simulink model "chris_3R_setpoint"  (R2024b)
settings: Solver=FixedStepDiscrete  StartTime=0.0  StopTime=3  FixedStep=0.1  MaxStep=0.1  RelTol=1e-3
libraries: simulink x1, realtime_pacer_lib x1
settings Model: Creator=RSL  LastModifiedBy=cwaight
settings SolverCC: AlgebraicLoopSolver=TrustRegion
settings DataIOCC: ReturnWorkspaceOutputs=off
settings DebuggingCC: UnconnectedInputMsg=warning  UnconnectedOutputMsg=warning  UnconnectedLineMsg=warning  ArithmeticOperatorsInVariantConditions=warning
settings ModelReferenceCC: EnableRefExpFcnMdlSchedulingChecks=on
settings SFSimCC: SimUseLocalCustomCode=off  CustomCodeUndefinedFunction=UseInterfaceOnly
settings RTWCC: RTWUseLocalCustomCode=off  GPUComputeCapability=3.5
settings CodeAppCC: StateflowObjectComments=on

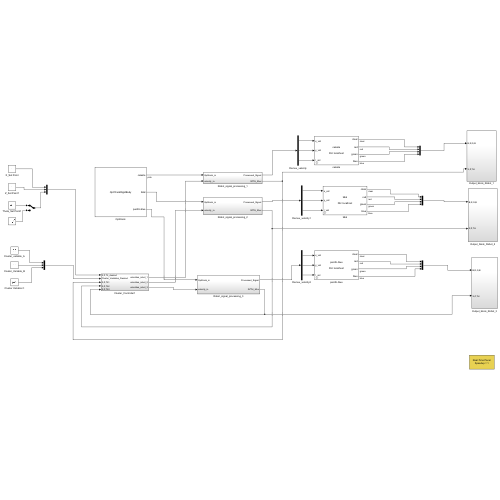
[thumbnail: Simulink's stored preview of the top-level diagram]
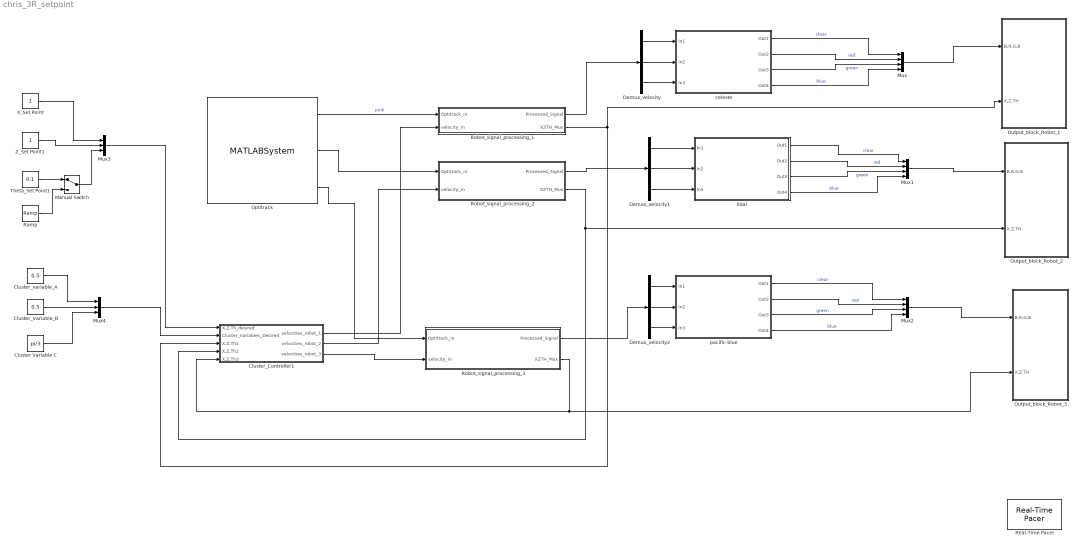
== system chris_3R_setpoint ==
  Cluster Variable C : Constant  Value=pi/3
  Cluster_Controller1 : Subsystem
  Cluster_Variable_B : Constant  Value=0.5
  Cluster_variable_A : Constant  Value=0.5
  Demux_velocity : Demux  Outputs=3
  Demux_velocity1 : Demux  Outputs=3
  Demux_velocity2 : Demux  Outputs=3
  Manual Switch : ManualSwitch
  Mux : Mux
  Mux1 : Mux
  Mux2 : Mux
  Mux3 : Mux  Inputs=3
  Mux4 : Mux  Inputs=3
  Optitrack : MATLABSystem  System=OptiTrackRigidBody  coordinateTransformationMatrix=[ 1, 0, 0; 0, 0, 1; 0, -1, 0 ]  rigidBodyNames={ 'celeste','tidal','pacific-blue'}  orientationFormat=Euler angles  debug=on  natNetHostAddress=127.0.0.1  natNetClientAddress=127.0.0.1  dllPath=C:\DecaMATLAB\NatNetSDK\lib\x64\NatNetML.dll  unicast=off
      mask Type: OptiTrackRigidBody
      mask Display:
      | disp('OptiTrackRigidBody');
      | port_label('output',1,'celeste');
      | port_label('output',2,'tidal');
      | port_label('output',3,'pacific-blue');
  Output_block_Robot_1 : Subsystem
  Output_block_Robot_2 : Subsystem
  Output_block_Robot_3 : Subsystem
  Ramp : simulink/Sources/Ramp  slope=1  start=0  InitialOutput=0.1
  Real-Time Pacer : realtime_pacer_lib/Real-Time Pacer  simTimePerRealTime=1
  Robot_signal_processing_1 : Subsystem
  Robot_signal_processing_2 : Subsystem
  Robot_signal_processing_3 : Subsystem
  "Theta_Set Point1 " : Constant  Value=0.1
  X_Set Point : Constant
  Z_Set Point1 : Constant
  celeste : Subsystem  mask(DecabotMask){robotName=celeste, decabotHelper=localhost, robotAddress=, useDataTurbine=off, useDirectSocket=on, debug=off}
      mask prompts: robotName "Robot name:"; decabotHelper "DecabotHelper/DataTurbine server:"; robotAddress "Robot network address (optional):"; useDataTurbine "Use DataTurbine"; useDirectSocket "Use direct robot TCP connection"; debug "Log debug messages"
      mask help: This is a masked subsystem that contains a Decabot block for bidirectional communication with a decabot over a direct TCP socket connection.
      mask init:
      | robotName = 'Nobody';
      | decabotHelper = 'localhost';
      | robotAddress = '';
      | useDataTurbine = true;
      | debug = true;
      mask TypeOptions robotName: decabot/robotName
      mask Callback robotName:
      | try
      |     set_param( gcb( ), 'Name', get_param( gcb( ), 'robotName' ) );
      | end
      mask TypeOptions decabotHelper: decabot/decabotHelper
      mask TypeOptions robotAddress: decabot/robotAddress
      mask TypeOptions useDataTurbine: decabot/useDataTurbine
      mask TypeOptions useDirectSocket: decabot/useDirectSocket
      mask TypeOptions debug: decabot/debug
      mask Display:
      | disp( [get_param( gcb( ), 'robotName' ) '\n\nDH: ' get_param( gcb( ), 'decabotHelper' ) ] );
      | 
      | port_label('input',1,'x_vel');
      | port_label('input',2,'y_vel');
      | port_label('input',3,'t_vel');
      | 
      | port_label('output',1,'clear');
      | port_label('output',2,'red');
      | port_label('output',3,'green');
      | port_label('output',4,'blue');
  pacific-blue : Subsystem  mask(DecabotMask){robotName=pacific-blue, decabotHelper=localhost, robotAddress=, useDataTurbine=off, useDirectSocket=on, debug=off}
      mask prompts: robotName "Robot name:"; decabotHelper "DecabotHelper/DataTurbine server:"; robotAddress "Robot network address (optional):"; useDataTurbine "Use DataTurbine"; useDirectSocket "Use direct robot TCP connection"; debug "Log debug messages"
      mask help: This is a masked subsystem that contains a Decabot block for bidirectional communication with a decabot over a direct TCP socket connection.
      mask init:
      | robotName = 'Nobody';
      | decabotHelper = 'localhost';
      | robotAddress = '';
      | useDataTurbine = true;
      | debug = true;
      mask TypeOptions robotName: decabot/robotName
      mask Callback robotName:
      | try
      |     set_param( gcb( ), 'Name', get_param( gcb( ), 'robotName' ) );
      | end
      mask TypeOptions decabotHelper: decabot/decabotHelper
      mask TypeOptions robotAddress: decabot/robotAddress
      mask TypeOptions useDataTurbine: decabot/useDataTurbine
      mask TypeOptions useDirectSocket: decabot/useDirectSocket
      mask TypeOptions debug: decabot/debug
      mask Display:
      | disp( [get_param( gcb( ), 'robotName' ) '\n\nDH: ' get_param( gcb( ), 'decabotHelper' ) ] );
      | 
      | port_label('input',1,'x_vel');
      | port_label('input',2,'y_vel');
      | port_label('input',3,'t_vel');
      | 
      | port_label('output',1,'clear');
      | port_label('output',2,'red');
      | port_label('output',3,'green');
      | port_label('output',4,'blue');
  tidal : Subsystem  mask(DecabotMask){robotName=tidal, decabotHelper=localhost, robotAddress=, useDataTurbine=off, useDirectSocket=on, debug=off}
      mask prompts: robotName "Robot name:"; decabotHelper "DecabotHelper/DataTurbine server:"; robotAddress "Robot network address (optional):"; useDataTurbine "Use DataTurbine"; useDirectSocket "Use direct robot TCP connection"; debug "Log debug messages"
      mask help: This is a masked subsystem that contains a Decabot block for bidirectional communication with a decabot over a direct TCP socket connection.
      mask init:
      | robotName = 'Nobody';
      | decabotHelper = 'localhost';
      | robotAddress = '';
      | useDataTurbine = true;
      | debug = true;
      mask TypeOptions robotName: decabot/robotName
      mask Callback robotName:
      | try
      |     set_param( gcb( ), 'Name', get_param( gcb( ), 'robotName' ) );
      | end
      mask TypeOptions decabotHelper: decabot/decabotHelper
      mask TypeOptions robotAddress: decabot/robotAddress
      mask TypeOptions useDataTurbine: decabot/useDataTurbine
      mask TypeOptions useDirectSocket: decabot/useDirectSocket
      mask TypeOptions debug: decabot/debug
      mask Display:
      | disp( [get_param( gcb( ), 'robotName' ) '\n\nDH: ' get_param( gcb( ), 'decabotHelper' ) ] );
      | 
      | port_label('input',1,'x_vel');
      | port_label('input',2,'y_vel');
      | port_label('input',3,'t_vel');
      | 
      | port_label('output',1,'clear');
      | port_label('output',2,'red');
      | port_label('output',3,'green');
      | port_label('output',4,'blue');
  wires:
  Demux_velocity/3 -> celeste/3(In3)
  Demux_velocity/1 -> celeste/1(In1)
  Demux_velocity/2 -> celeste/2(In2)
  X_Set Point/1 -> Mux3/1
  Optitrack/1 -> Robot_signal_processing_1/1(Optitrack_in)  "pink"
  Robot_signal_processing_1/1(Processed_Signal) -> Demux_velocity/1
  celeste/1(Out1) -> Mux/1  "clear"
  celeste/2(Out2) -> Mux/2  "red"
  celeste/3(Out3) -> Mux/3  "green"
  celeste/4(Out4) -> Mux/4  "blue"
  Robot_signal_processing_1/2(XZTH_Mux) -> Output_block_Robot_1/2(X,Z,TH), Cluster_Controller1/3(X,Z,Th1)
  Mux/1 -> Output_block_Robot_1/1(B,R,G,B)
  Demux_velocity1/3 -> tidal/3(In3)
  Demux_velocity1/1 -> tidal/1(In1)
  Demux_velocity1/2 -> tidal/2(In2)
  Robot_signal_processing_2/1(Processed_Signal) -> Demux_velocity1/1
  tidal/1(Out1) -> Mux1/1  "clear"
  tidal/2(Out2) -> Mux1/2  "red"
  tidal/3(Out3) -> Mux1/3  "green"
  tidal/4(Out4) -> Mux1/4  "blue"
  Mux1/1 -> Output_block_Robot_2/1(B,R,G,B)
  Demux_velocity2/3 -> pacific-blue/3(In3)
  Demux_velocity2/1 -> pacific-blue/1(In1)
  Demux_velocity2/2 -> pacific-blue/2(In2)
  Robot_signal_processing_3/1(Processed_Signal) -> Demux_velocity2/1
  pacific-blue/1(Out1) -> Mux2/1  "clear"
  pacific-blue/2(Out2) -> Mux2/2  "red"
  pacific-blue/3(Out3) -> Mux2/3  "green"
  pacific-blue/4(Out4) -> Mux2/4  "blue"
  Mux2/1 -> Output_block_Robot_3/1(B,R,G,B)
  Robot_signal_processing_3/2(XZTH_Mux) -> Output_block_Robot_3/2(X,Z,TH), Cluster_Controller1/5(X,Z,Th3)
  Optitrack/2 -> Robot_signal_processing_2/1(Optitrack_in)
  Optitrack/3 -> Robot_signal_processing_3/1(Optitrack_in)
  Cluster_Controller1/1(velocities_robot_1) -> Robot_signal_processing_1/2(velocity_in)
  Z_Set Point1/1 -> Mux3/2
  Cluster_Controller1/3(velocities_robot_3) -> Robot_signal_processing_3/2(velocity_in)
  Mux3/1 -> Cluster_Controller1/1(X,Z,Th_desired)
  Cluster_Controller1/2(velocities_robot_2) -> Robot_signal_processing_2/2(velocity_in)
  Cluster_variable_A/1 -> Mux4/1
  Cluster_Variable_B/1 -> Mux4/2
  Cluster Variable C/1 -> Mux4/3
  Mux4/1 -> Cluster_Controller1/2(Cluster_Variables_Desired)
  Robot_signal_processing_2/2(XZTH_Mux) -> Cluster_Controller1/4(X,Z,Th2), Output_block_Robot_2/2(X,Z,TH)
  Ramp/1 -> Manual Switch/2
  "Theta_Set Point1 "/1 -> Manual Switch/1
  Manual Switch/1 -> Mux3/3

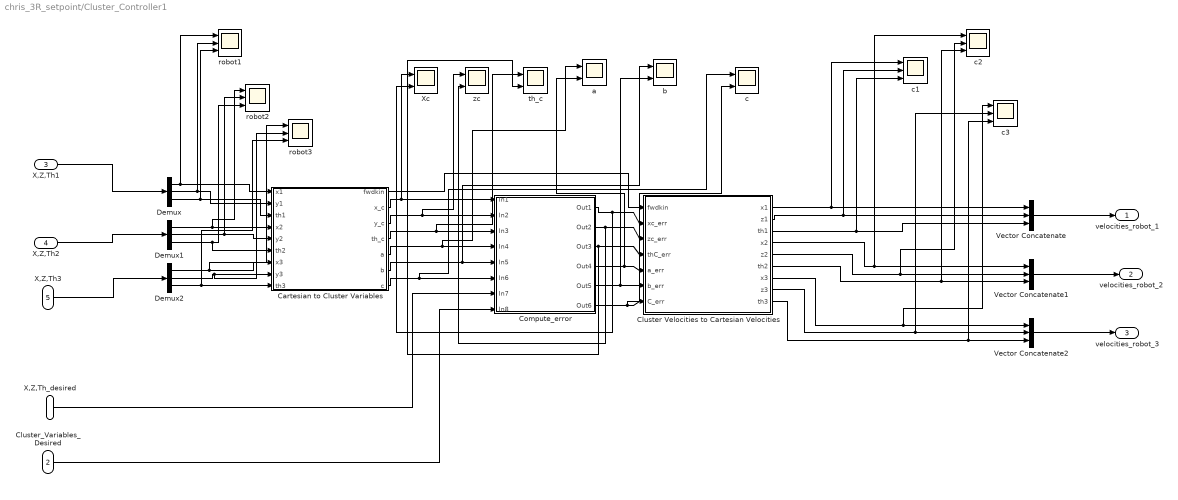
== system chris_3R_setpoint/Cluster_Controller1 ==
  X,Z,Th_desired : Inport
  Cluster_Variables_Desired : Inport  Port=2
  X,Z,Th1 : Inport  Port=3
  X,Z,Th2 : Inport  Port=4
  X,Z,Th3 : Inport  Port=5
  Cartesian to Cluster Variables : MATLAB Function  TreatAsAtomicUnit=on
  Cluster Velocities to Cartesian Velocities : MATLAB Function  TreatAsAtomicUnit=on
  Compute_error : Subsystem
  Demux : Demux  Outputs=3
  Demux1 : Demux  Outputs=3
  Demux2 : Demux  Outputs=3
  Vector Concatenate : Concatenate  NumInputs=3
  Vector Concatenate1 : Concatenate  NumInputs=3
  Vector Concatenate2 : Concatenate  NumInputs=3
  Xc : Scope  NumInputPorts=2
  a : Scope  NumInputPorts=2
  b : Scope  NumInputPorts=2
  c : Scope  NumInputPorts=2
  c1 : Scope  NumInputPorts=3
  c2 : Scope  NumInputPorts=3
  c3 : Scope  NumInputPorts=3
  robot1 : Scope  NumInputPorts=3
  robot2 : Scope  NumInputPorts=3
  robot3 : Scope  NumInputPorts=3
  th_c : Scope  NumInputPorts=2
  zc : Scope  NumInputPorts=2
  velocities_robot_1 : Outport
  velocities_robot_2 : Outport  Port=2
  velocities_robot_3 : Outport  Port=3
  wires:
  X,Z,Th1/1 -> Demux/1
  X,Z,Th2/1 -> Demux1/1
  X,Z,Th3/1 -> Demux2/1
  Vector Concatenate/1 -> velocities_robot_1/1
  Cluster Velocities to Cartesian Velocities/2(z1) -> c1/2, Vector Concatenate/2
  Cluster Velocities to Cartesian Velocities/1(x1) -> c1/1, Vector Concatenate/1
  Vector Concatenate1/1 -> velocities_robot_2/1
  Cluster Velocities to Cartesian Velocities/5(z2) -> c2/2, Vector Concatenate1/2
  Cluster Velocities to Cartesian Velocities/4(x2) -> c2/1, Vector Concatenate1/1
  Vector Concatenate2/1 -> velocities_robot_3/1
  Cluster Velocities to Cartesian Velocities/8(z3) -> c3/2, Vector Concatenate2/2
  Cluster Velocities to Cartesian Velocities/7(x3) -> c3/1, Vector Concatenate2/1
  Demux/1 -> robot1/1, Cartesian to Cluster Variables/1(x1)
  Demux/2 -> robot1/2, Cartesian to Cluster Variables/2(y1)
  Demux/3 -> robot1/3, Cartesian to Cluster Variables/3(th1)
  Demux1/1 -> robot2/1, Cartesian to Cluster Variables/4(x2)
  Demux1/2 -> robot2/2, Cartesian to Cluster Variables/5(y2)
  Demux1/3 -> robot2/3, Cartesian to Cluster Variables/6(th2)
  Demux2/1 -> robot3/1, Cartesian to Cluster Variables/7(x3)
  Demux2/2 -> robot3/2, Cartesian to Cluster Variables/8(y3)
  Demux2/3 -> robot3/3, Cartesian to Cluster Variables/9(th3)
  Cartesian to Cluster Variables/2(x_c) -> Xc/1, Compute_error/1(In1)
  Cartesian to Cluster Variables/3(y_c) -> zc/1, Compute_error/2(In2)
  Cartesian to Cluster Variables/4(th_c) -> th_c/1, Compute_error/3(In3)
  Cartesian to Cluster Variables/5(a) -> a/1, Compute_error/4(In4)
  Cartesian to Cluster Variables/6(b) -> b/1, Compute_error/5(In5)
  Cartesian to Cluster Variables/7(c) -> c/1, Compute_error/6(In6)
  X,Z,Th_desired/1 -> Compute_error/7(In7)
  Cluster_Variables_Desired/1 -> Compute_error/8(In8)
  Compute_error/1(Out1) -> Xc/2, Cluster Velocities to Cartesian Velocities/2(xc_err)
  Compute_error/2(Out2) -> zc/2, Cluster Velocities to Cartesian Velocities/3(zc_err)
  Compute_error/3(Out3) -> th_c/2, Cluster Velocities to Cartesian Velocities/4(thC_err)
  Compute_error/4(Out4) -> a/2, Cluster Velocities to Cartesian Velocities/5(a_err)
  Compute_error/5(Out5) -> b/2, Cluster Velocities to Cartesian Velocities/6(b_err)
  Compute_error/6(Out6) -> c/2, Cluster Velocities to Cartesian Velocities/7(C_err)
  Cartesian to Cluster Variables/1(fwdkin) -> Cluster Velocities to Cartesian Velocities/1(fwdkin)
  Cluster Velocities to Cartesian Velocities/3(th1) -> c1/3, Vector Concatenate/3
  Cluster Velocities to Cartesian Velocities/6(th2) -> c2/3, Vector Concatenate1/3
  Cluster Velocities to Cartesian Velocities/9(th3) -> c3/3, Vector Concatenate2/3

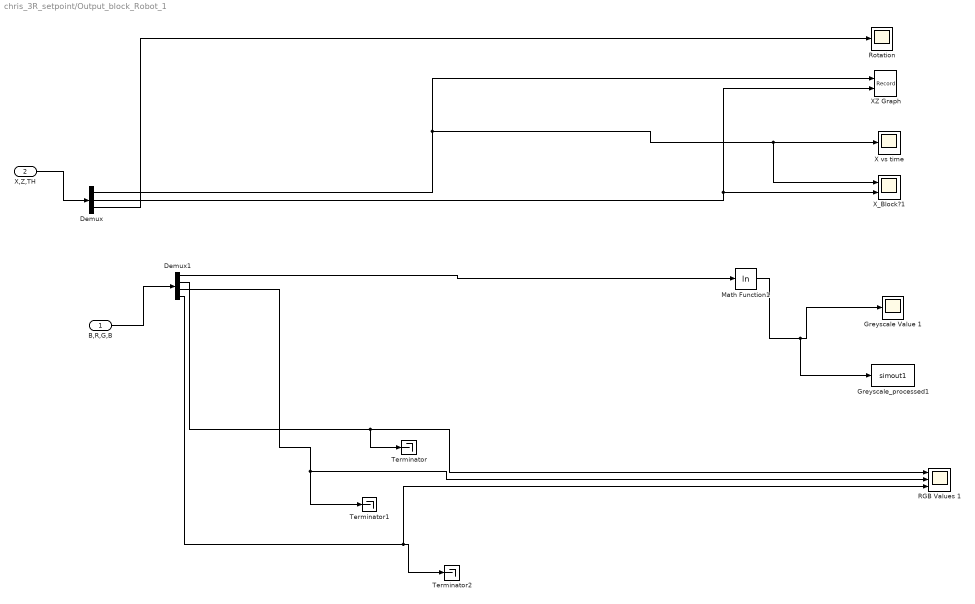
== system chris_3R_setpoint/Output_block_Robot_1 ==
  B,R,G,B : Inport
  X,Z,TH : Inport  Port=2
  " Greyscale_processed1" : ToWorkspace  VariableName=simout1  SaveFormat=Timeseries  SampleTime=-1
  Demux : Demux  Outputs=3
  Demux1 : Demux
  Greyscale Value 1 : Scope
  Math Function1 : Math  Operator=log  SignedPower=on
  "RGB Values 1 " : Scope  NumInputPorts=3
  Rotation : Scope
  Terminator : Terminator
  Terminator1 : Terminator
  Terminator2 : Terminator
  X vs time : Scope
  XZ Graph : Record  FileSettingsInternal="{\"entries\":[{\"content\":{\"excelSettings\":{\"content\":{},\"type\":\"Streamout.ExcelSettings\"}},\"type\":\"Streamout.FileSettingStorage\",\"uuid\":\"\"}],\"packageUris\":[\"http:\\/\\/schema.mathworks.com\\/mf0\\/streamout_blocks\\/R2020a\"],\"version\":\"1.0\"}"  Layout=[1 1]  SignalsInternal="{\"entries\":[{\"content\":{\"signals\":[{\"content\":{\"blockPath\":[],\"dimensions\":[1],\"domain\":\"\",\"lineColor\":\"#a2142f\",\"plots\":[ 1 ],\"port\":1,\"sid\":[\"\"],\"signalID\":1,\"signalName\":\"Demux:1\"},\"type\":\"RecordBlkView.Signal\",\"uuid\":\"\"},{\"content\":{\"blockPath\":[],\"dimensions\":[1],\"domain\":\"\",\"lineColor\":\"#139fff\",\"plots\":[ 1 ],\"port\":2,\"sid\":[\"\"],\"signalID\":2,\"signalName\":\"Demux:2\"},\"type\":\"RecordBlkView.Signal\",\"uuid\":\"\"}]},\"type\":\"RecordBlkView.InputSignals\",\"uuid\":\"\"}],\"packageUris\":[\"http:\\/\\/schema.mathworks.com\\/mf0\\/streamout_blocks\\/R2020a\"],\"version\":\"1.0\"}"  VisualizationBindings="{\"xyplotplugin\":{\"info\":[{\"series\":[{\"bindingParametersList\":[{\"parameter\":\"X-Axis\",\"signalID\":1,\"signalName\":\"Demux:1\"},{\"parameter\":\"Y-Axis\",\"signalID\":2,\"signalName\":\"Demux:2\"}],\"seriesID\":0}],\"subplotID\":1}]}}"  CompatibilityTag=XY  st=-1
  X_Block?1 : Scope  NumInputPorts=2
  wires:
  Demux/3 -> Rotation/1
  Demux/2 -> XZ Graph/2, X_Block?1/2
  Demux1/2 -> "RGB Values 1 "/1, Terminator/1
  Demux1/4 -> "RGB Values 1 "/3, Terminator2/1
  Math Function1/1 -> " Greyscale_processed1"/1, Greyscale Value 1/1
  Demux1/3 -> Terminator1/1, "RGB Values 1 "/2
  X,Z,TH/1 -> Demux/1
  Demux/1 -> X_Block?1/1, X vs time/1, XZ Graph/1
  Demux1/1 -> Math Function1/1
  B,R,G,B/1 -> Demux1/1

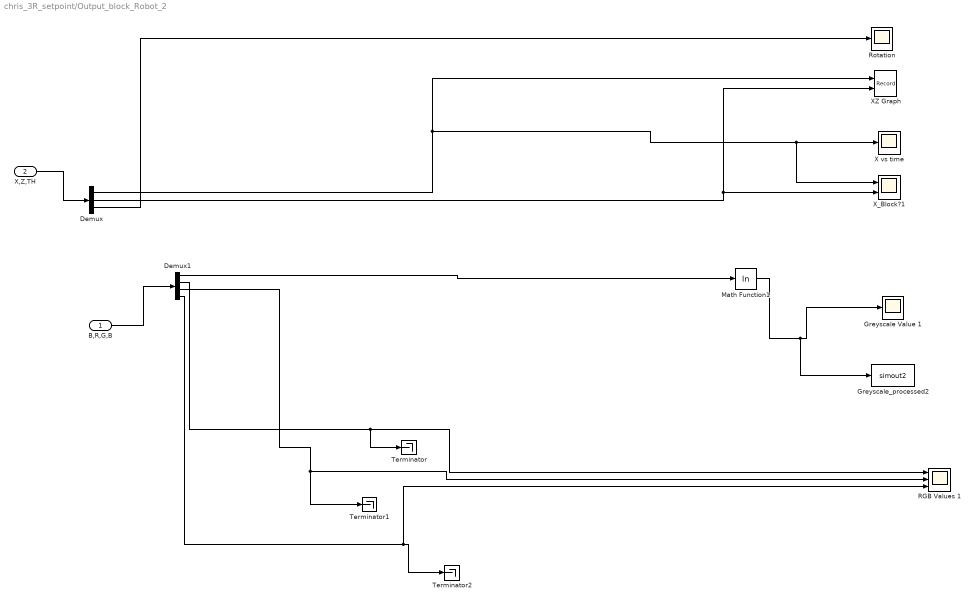
== system chris_3R_setpoint/Output_block_Robot_2 ==
  B,R,G,B : Inport
  X,Z,TH : Inport  Port=2
  " Greyscale_processed2" : ToWorkspace  VariableName=simout2  SaveFormat=Timeseries  SampleTime=-1
  Demux : Demux  Outputs=3
  Demux1 : Demux
  Greyscale Value 1 : Scope
  Math Function1 : Math  Operator=log  SignedPower=on
  "RGB Values 1 " : Scope  NumInputPorts=3
  Rotation : Scope
  Terminator : Terminator
  Terminator1 : Terminator
  Terminator2 : Terminator
  X vs time : Scope
  XZ Graph : Record  FileSettingsInternal="{\"entries\":[{\"content\":{\"excelSettings\":{\"content\":{},\"type\":\"Streamout.ExcelSettings\"}},\"type\":\"Streamout.FileSettingStorage\",\"uuid\":\"\"}],\"packageUris\":[\"http:\\/\\/schema.mathworks.com\\/mf0\\/streamout_blocks\\/R2020a\"],\"version\":\"1.0\"}"  Layout=[1 1]  SignalsInternal="{\"entries\":[{\"content\":{\"signals\":[{\"content\":{\"blockPath\":[],\"dimensions\":[1],\"domain\":\"\",\"lineColor\":\"#a2142f\",\"plots\":[ 1 ],\"port\":1,\"sid\":[\"\"],\"signalID\":1,\"signalName\":\"Demux:1\"},\"type\":\"RecordBlkView.Signal\",\"uuid\":\"\"},{\"content\":{\"blockPath\":[],\"dimensions\":[1],\"domain\":\"\",\"lineColor\":\"#139fff\",\"plots\":[ 1 ],\"port\":2,\"sid\":[\"\"],\"signalID\":2,\"signalName\":\"Demux:2\"},\"type\":\"RecordBlkView.Signal\",\"uuid\":\"\"}]},\"type\":\"RecordBlkView.InputSignals\",\"uuid\":\"\"}],\"packageUris\":[\"http:\\/\\/schema.mathworks.com\\/mf0\\/streamout_blocks\\/R2020a\"],\"version\":\"1.0\"}"  VisualizationBindings="{\"xyplotplugin\":{\"info\":[{\"series\":[{\"bindingParametersList\":[{\"parameter\":\"X-Axis\",\"signalID\":1,\"signalName\":\"Demux:1\"},{\"parameter\":\"Y-Axis\",\"signalID\":2,\"signalName\":\"Demux:2\"}],\"seriesID\":0}],\"subplotID\":1}]}}"  CompatibilityTag=XY  st=-1
  X_Block?1 : Scope  NumInputPorts=2
  wires:
  Demux/3 -> Rotation/1
  Demux/2 -> XZ Graph/2, X_Block?1/2
  Demux1/2 -> "RGB Values 1 "/1, Terminator/1
  Demux1/4 -> "RGB Values 1 "/3, Terminator2/1
  Math Function1/1 -> " Greyscale_processed2"/1, Greyscale Value 1/1
  Demux1/3 -> Terminator1/1, "RGB Values 1 "/2
  X,Z,TH/1 -> Demux/1
  Demux/1 -> X_Block?1/1, X vs time/1, XZ Graph/1
  Demux1/1 -> Math Function1/1
  B,R,G,B/1 -> Demux1/1

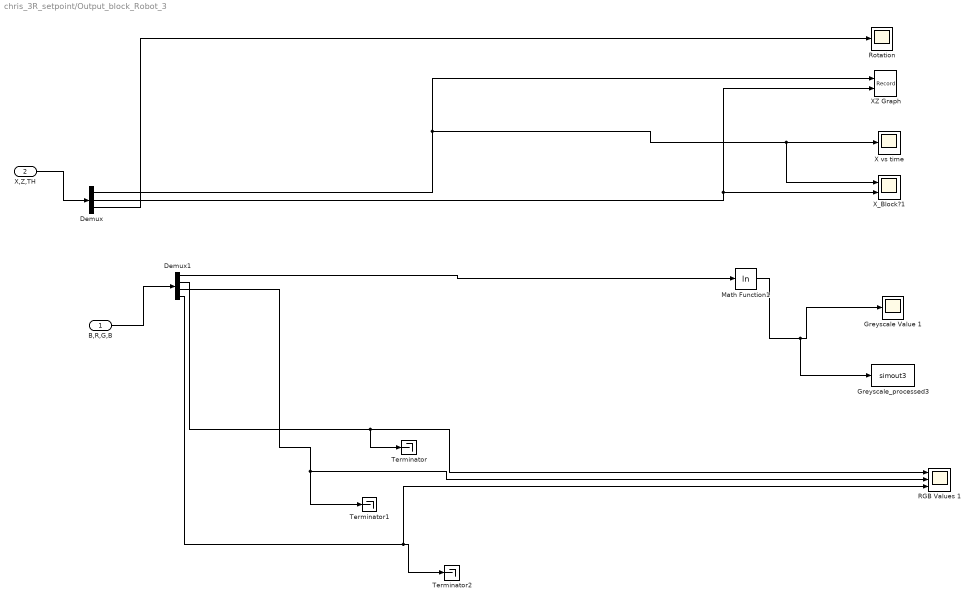
== system chris_3R_setpoint/Output_block_Robot_3 ==
  B,R,G,B : Inport
  X,Z,TH : Inport  Port=2
  " Greyscale_processed3" : ToWorkspace  VariableName=simout3  SaveFormat=Timeseries  SampleTime=-1
  Demux : Demux  Outputs=3
  Demux1 : Demux
  Greyscale Value 1 : Scope
  Math Function1 : Math  Operator=log  SignedPower=on
  "RGB Values 1 " : Scope  NumInputPorts=3
  Rotation : Scope
  Terminator : Terminator
  Terminator1 : Terminator
  Terminator2 : Terminator
  X vs time : Scope
  XZ Graph : Record  FileSettingsInternal="{\"entries\":[{\"content\":{\"excelSettings\":{\"content\":{},\"type\":\"Streamout.ExcelSettings\"}},\"type\":\"Streamout.FileSettingStorage\",\"uuid\":\"\"}],\"packageUris\":[\"http:\\/\\/schema.mathworks.com\\/mf0\\/streamout_blocks\\/R2020a\"],\"version\":\"1.0\"}"  Layout=[1 1]  SignalsInternal="{\"entries\":[{\"content\":{\"signals\":[{\"content\":{\"blockPath\":[],\"dimensions\":[1],\"domain\":\"\",\"lineColor\":\"#a2142f\",\"plots\":[ 1 ],\"port\":1,\"sid\":[\"\"],\"signalID\":1,\"signalName\":\"Demux:1\"},\"type\":\"RecordBlkView.Signal\",\"uuid\":\"\"},{\"content\":{\"blockPath\":[],\"dimensions\":[1],\"domain\":\"\",\"lineColor\":\"#139fff\",\"plots\":[ 1 ],\"port\":2,\"sid\":[\"\"],\"signalID\":2,\"signalName\":\"Demux:2\"},\"type\":\"RecordBlkView.Signal\",\"uuid\":\"\"}]},\"type\":\"RecordBlkView.InputSignals\",\"uuid\":\"\"}],\"packageUris\":[\"http:\\/\\/schema.mathworks.com\\/mf0\\/streamout_blocks\\/R2020a\"],\"version\":\"1.0\"}"  VisualizationBindings="{\"xyplotplugin\":{\"info\":[{\"series\":[{\"bindingParametersList\":[{\"parameter\":\"X-Axis\",\"signalID\":1,\"signalName\":\"Demux:1\"},{\"parameter\":\"Y-Axis\",\"signalID\":2,\"signalName\":\"Demux:2\"}],\"seriesID\":0}],\"subplotID\":1}]}}"  CompatibilityTag=XY  st=-1
  X_Block?1 : Scope  NumInputPorts=2
  wires:
  Demux/3 -> Rotation/1
  Demux/2 -> XZ Graph/2, X_Block?1/2
  Demux1/2 -> "RGB Values 1 "/1, Terminator/1
  Demux1/4 -> "RGB Values 1 "/3, Terminator2/1
  Math Function1/1 -> " Greyscale_processed3"/1, Greyscale Value 1/1
  Demux1/3 -> Terminator1/1, "RGB Values 1 "/2
  X,Z,TH/1 -> Demux/1
  Demux/1 -> X_Block?1/1, X vs time/1, XZ Graph/1
  Demux1/1 -> Math Function1/1
  B,R,G,B/1 -> Demux1/1

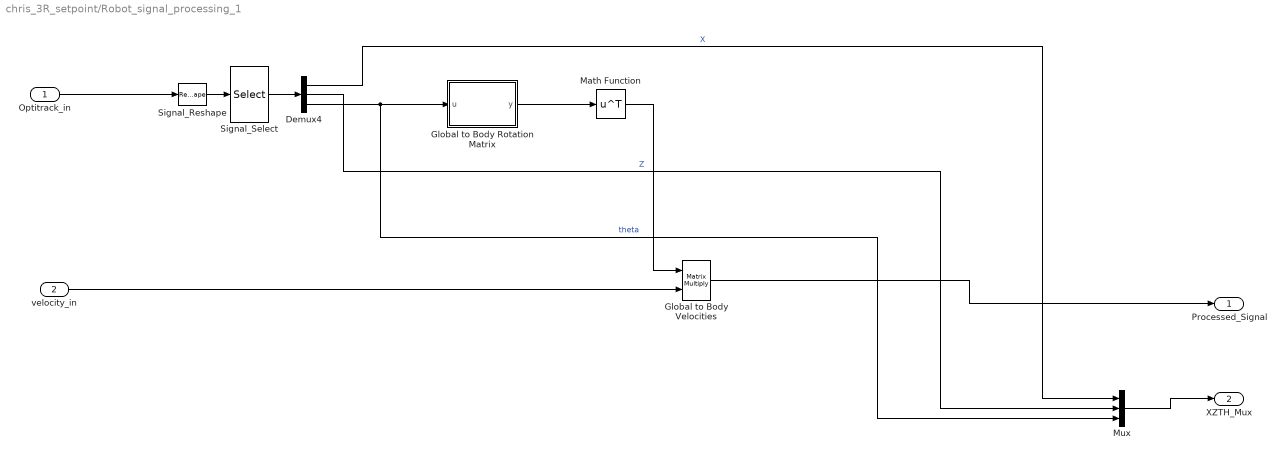
== system chris_3R_setpoint/Robot_signal_processing_1 ==
  Optitrack_in : Inport
  velocity_in : Inport  Port=2
  Demux4 : Demux  Outputs=3
  Global to Body Velocities : Product  Multiplication=Matrix(*)
  Global to Body Rotation Matrix : MATLAB Function  TreatAsAtomicUnit=on
  Math Function : Math  Operator=transpose  SignedPower=on
  Mux : Mux  Inputs=3
  Signal_Reshape : Reshape  OutputDimensions=6
  Signal_Select : Selector  InputPortWidth=6  IndexOptions=Index vector (dialog)  Indices=[1 2 6]  OutputSizes=1
  Processed_Signal : Outport
  XZTH_Mux : Outport  Port=2
  wires:
  Demux4/1 -> Mux/1  "X"
  Demux4/3 -> Mux/3, Global to Body Rotation Matrix/1(u)  "theta"
  Demux4/2 -> Mux/2  "Z"
  Global to Body Velocities/1 -> Processed_Signal/1
  Signal_Reshape/1 -> Signal_Select/1
  velocity_in/1 -> Global to Body Velocities/2
  Optitrack_in/1 -> Signal_Reshape/1
  Global to Body Rotation Matrix/1(y) -> Math Function/1
  Signal_Select/1 -> Demux4/1
  Math Function/1 -> Global to Body Velocities/1
  Mux/1 -> XZTH_Mux/1

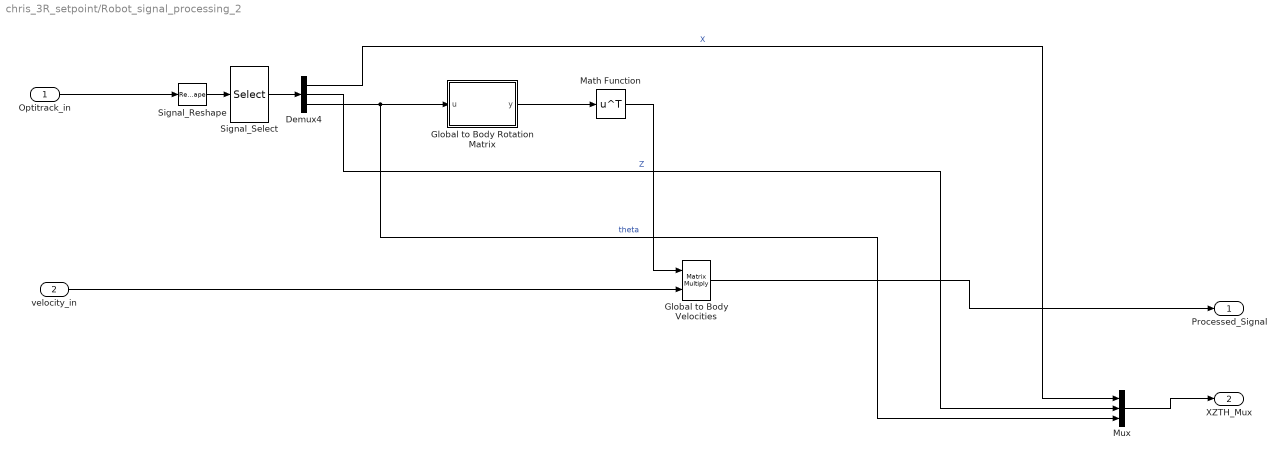
== system chris_3R_setpoint/Robot_signal_processing_2 ==
  Optitrack_in : Inport
  velocity_in : Inport  Port=2
  Demux4 : Demux  Outputs=3
  Global to Body Velocities : Product  Multiplication=Matrix(*)
  Global to Body Rotation Matrix : MATLAB Function  TreatAsAtomicUnit=on
  Math Function : Math  Operator=transpose  SignedPower=on
  Mux : Mux  Inputs=3
  Signal_Reshape : Reshape  OutputDimensions=6
  Signal_Select : Selector  InputPortWidth=6  IndexOptions=Index vector (dialog)  Indices=[1 2 6]  OutputSizes=1
  Processed_Signal : Outport
  XZTH_Mux : Outport  Port=2
  wires:
  Demux4/1 -> Mux/1  "X"
  Demux4/3 -> Mux/3, Global to Body Rotation Matrix/1(u)  "theta"
  Demux4/2 -> Mux/2  "Z"
  Global to Body Velocities/1 -> Processed_Signal/1
  Signal_Reshape/1 -> Signal_Select/1
  velocity_in/1 -> Global to Body Velocities/2
  Optitrack_in/1 -> Signal_Reshape/1
  Global to Body Rotation Matrix/1(y) -> Math Function/1
  Signal_Select/1 -> Demux4/1
  Math Function/1 -> Global to Body Velocities/1
  Mux/1 -> XZTH_Mux/1

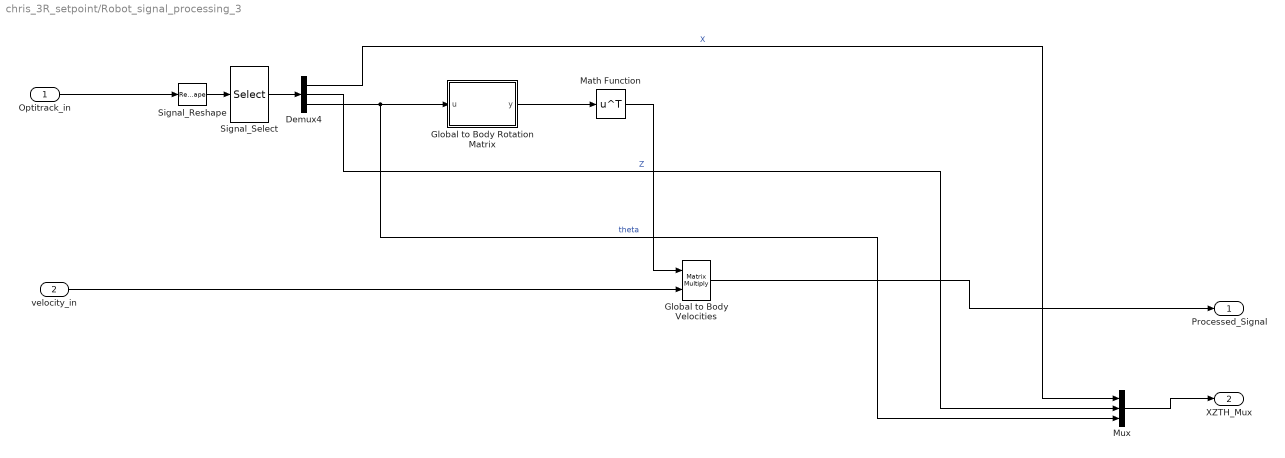
== system chris_3R_setpoint/Robot_signal_processing_3 ==
  Optitrack_in : Inport
  velocity_in : Inport  Port=2
  Demux4 : Demux  Outputs=3
  Global to Body Velocities : Product  Multiplication=Matrix(*)
  Global to Body Rotation Matrix : MATLAB Function  TreatAsAtomicUnit=on
  Math Function : Math  Operator=transpose  SignedPower=on
  Mux : Mux  Inputs=3
  Signal_Reshape : Reshape  OutputDimensions=6
  Signal_Select : Selector  InputPortWidth=6  IndexOptions=Index vector (dialog)  Indices=[1 2 6]  OutputSizes=1
  Processed_Signal : Outport
  XZTH_Mux : Outport  Port=2
  wires:
  Demux4/1 -> Mux/1  "X"
  Demux4/3 -> Mux/3, Global to Body Rotation Matrix/1(u)  "theta"
  Demux4/2 -> Mux/2  "Z"
  Global to Body Velocities/1 -> Processed_Signal/1
  Signal_Reshape/1 -> Signal_Select/1
  velocity_in/1 -> Global to Body Velocities/2
  Optitrack_in/1 -> Signal_Reshape/1
  Global to Body Rotation Matrix/1(y) -> Math Function/1
  Signal_Select/1 -> Demux4/1
  Math Function/1 -> Global to Body Velocities/1
  Mux/1 -> XZTH_Mux/1

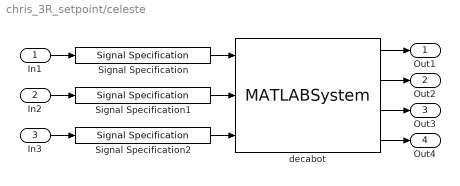
== system chris_3R_setpoint/celeste ==
  In1 : Inport
  In2 : Inport  Port=2
  In3 : Inport  Port=3
  Signal Specification : SignalSpecification  OutDataTypeStr=double  Dimensions=1
  Signal Specification1 : SignalSpecification  OutDataTypeStr=double  Dimensions=1
  Signal Specification2 : SignalSpecification  OutDataTypeStr=double  Dimensions=1
  decabot : MATLABSystem  System=Decabot  robotName=celeste  decabotHelper=localhost  useDataTurbine=off  useDirectSocket=on  debug=off
      mask Type: Decabot
      mask Display:
      | disp('celeste\n\nDH: localhost');
      | port_label('input',1,'x_vel');
      | port_label('input',2,'y_vel');
      | port_label('input',3,'t_vel');
      | port_label('output',1,'clear');
      | port_label('output',2,'red');
      | port_label('output',3,'green');
      | port_label('output',4,'blue');
  Out1 : Outport
  Out2 : Outport  Port=2
  Out3 : Outport  Port=3
  Out4 : Outport  Port=4
  wires:
  Signal Specification2/1 -> decabot/3
  Signal Specification1/1 -> decabot/2
  Signal Specification/1 -> decabot/1
  In2/1 -> Signal Specification1/1
  decabot/4 -> Out4/1
  decabot/1 -> Out1/1
  decabot/3 -> Out3/1
  decabot/2 -> Out2/1
  In1/1 -> Signal Specification/1
  In3/1 -> Signal Specification2/1

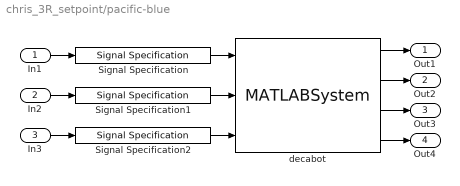
== system chris_3R_setpoint/pacific-blue ==
  In1 : Inport
  In2 : Inport  Port=2
  In3 : Inport  Port=3
  Signal Specification : SignalSpecification  OutDataTypeStr=double  Dimensions=1
  Signal Specification1 : SignalSpecification  OutDataTypeStr=double  Dimensions=1
  Signal Specification2 : SignalSpecification  OutDataTypeStr=double  Dimensions=1
  decabot : MATLABSystem  System=Decabot  robotName=pacific-blue  decabotHelper=localhost  useDataTurbine=off  useDirectSocket=on  debug=off
      mask Type: Decabot
      mask Display:
      | disp('pacific-blue\n\nDH: localhost');
      | port_label('input',1,'x_vel');
      | port_label('input',2,'y_vel');
      | port_label('input',3,'t_vel');
      | port_label('output',1,'clear');
      | port_label('output',2,'red');
      | port_label('output',3,'green');
      | port_label('output',4,'blue');
  Out1 : Outport
  Out2 : Outport  Port=2
  Out3 : Outport  Port=3
  Out4 : Outport  Port=4
  wires:
  Signal Specification2/1 -> decabot/3
  Signal Specification1/1 -> decabot/2
  Signal Specification/1 -> decabot/1
  In2/1 -> Signal Specification1/1
  decabot/4 -> Out4/1
  decabot/1 -> Out1/1
  decabot/3 -> Out3/1
  decabot/2 -> Out2/1
  In1/1 -> Signal Specification/1
  In3/1 -> Signal Specification2/1

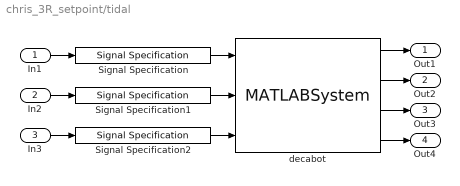
== system chris_3R_setpoint/tidal ==
  In1 : Inport
  In2 : Inport  Port=2
  In3 : Inport  Port=3
  Signal Specification : SignalSpecification  OutDataTypeStr=double  Dimensions=1
  Signal Specification1 : SignalSpecification  OutDataTypeStr=double  Dimensions=1
  Signal Specification2 : SignalSpecification  OutDataTypeStr=double  Dimensions=1
  decabot : MATLABSystem  System=Decabot  robotName=tidal  decabotHelper=localhost  useDataTurbine=off  useDirectSocket=on  debug=off
      mask Type: Decabot
      mask Display:
      | disp('tidal\n\nDH: localhost');
      | port_label('input',1,'x_vel');
      | port_label('input',2,'y_vel');
      | port_label('input',3,'t_vel');
      | port_label('output',1,'clear');
      | port_label('output',2,'red');
      | port_label('output',3,'green');
      | port_label('output',4,'blue');
  Out1 : Outport
  Out2 : Outport  Port=2
  Out3 : Outport  Port=3
  Out4 : Outport  Port=4
  wires:
  Signal Specification2/1 -> decabot/3
  Signal Specification1/1 -> decabot/2
  Signal Specification/1 -> decabot/1
  In2/1 -> Signal Specification1/1
  decabot/4 -> Out4/1
  decabot/1 -> Out1/1
  decabot/3 -> Out3/1
  decabot/2 -> Out2/1
  In1/1 -> Signal Specification/1
  In3/1 -> Signal Specification2/1

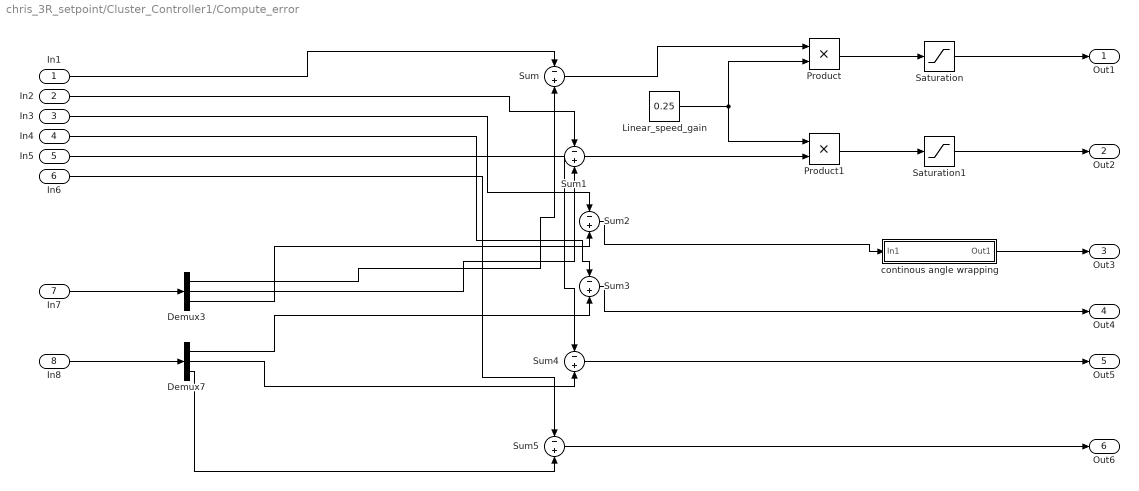
== system chris_3R_setpoint/Cluster_Controller1/Compute_error ==
  In1 : Inport
  In2 : Inport  Port=2
  In3 : Inport  Port=3
  In4 : Inport  Port=4
  In5 : Inport  Port=5
  In6 : Inport  Port=6
  In7 : Inport  Port=7
  In8 : Inport  Port=8
  Demux3 : Demux  Outputs=3
  Demux7 : Demux  Outputs=3
  Linear_speed_gain : Constant  Value=0.25
  Product : Product
  Product1 : Product
  Saturation : Saturate
  Saturation1 : Saturate
  Sum{,1..5} (6 alike) : Sum  Inputs=-+
  continous angle wrapping : Subsystem
  Out1 : Outport
  Out2 : Outport  Port=2
  Out3 : Outport  Port=3
  Out4 : Outport  Port=4
  Out5 : Outport  Port=5
  Out6 : Outport  Port=6
  wires:
  In3/1 -> Sum2/1
  Demux3/2 -> Sum1/2
  Sum3/1 -> Out4/1
  In2/1 -> Sum1/1
  Demux3/3 -> Sum2/2
  Demux7/3 -> Sum5/2
  In8/1 -> Demux7/1
  Demux7/1 -> Sum3/2
  In1/1 -> Sum/1
  In5/1 -> Sum4/1
  Demux7/2 -> Sum4/2
  In6/1 -> Sum5/1
  Sum4/1 -> Out5/1
  Sum5/1 -> Out6/1
  Demux3/1 -> Sum/2
  In4/1 -> Sum3/1
  In7/1 -> Demux3/1
  Sum2/1 -> continous angle wrapping/1(In1)
  continous angle wrapping/1(Out1) -> Out3/1
  Sum/1 -> Product/1
  Linear_speed_gain/1 -> Product/2, Product1/1
  Sum1/1 -> Product1/2
  Saturation/1 -> Out1/1
  Product/1 -> Saturation/1
  Product1/1 -> Saturation1/1
  Saturation1/1 -> Out2/1

== system chris_3R_setpoint/Cluster_Controller1/Compute_error/continous angle wrapping ==
  In1 : Inport
  Constant : Constant  Value=pi
  Constant1 : Constant  Value=2*pi
  Math Function : Math  Operator=mod  SignedPower=on
  Sum6 : Sum
  Sum7 : Sum  Inputs=-+
  Out1 : Outport
  wires:
  In1/1 -> Sum6/2
  Math Function/1 -> Sum7/2
  Constant/1 -> Sum7/1, Sum6/1
  Sum6/1 -> Math Function/1
  Constant1/1 -> Math Function/2
  Sum7/1 -> Out1/1

== matlab function chris_3R_setpoint/Robot_signal_processing_2/Global to Body Rotation Matrix ==
  data: u input; y output
function y = fcn(u)

y = [cos(u) -sin(u) 0; sin(u) cos(u) 0; 0 0 1];

== matlab function chris_3R_setpoint/Robot_signal_processing_3/Global to Body Rotation Matrix ==
  data: u input; y output
function y = fcn(u)

y = [cos(u) -sin(u) 0; sin(u) cos(u) 0; 0 0 1];

== matlab function chris_3R_setpoint/Cluster_Controller1/Cartesian to Cluster Variables ==
  data: fwdkin output; x1 input; x_c output; y1 input; th1 input; x2 input; y2 input; th2 input; x3 input; y3 input; th3 input; y_c output; th_c output; a output; b output; c output
function [fwdkin, x_c, y_c, th_c, a, b, c]   = Forward_Kinematics(x1, y1, th1, x2,y2,th2, x3,y3,th3)
% Centre frame
x_c = (x1+x2+x3)/3;
y_c = (y1+y2+y3)/3;
theta_c = atan2((2/3)*x1 - (1/3)*(x2 + x3), (2/3)*y1 - (1/3)*(y2 + y3));
% SAS Properties of triangle
p = sqrt((x1 - x2)^2 + (y1 - y2)^2);
q = sqrt((x3 - x1)^2 + (y1 - y3)^2);
beta = acos((p^2 + q^2 - (x3 - x2)^2 - (y3 - y2)^2) / (2*p*q));
% Rotation vectors
phi1 = th1 + theta_c;
phi2 = th2 + theta_c;
phi3 = th3 + theta_c;
a =p;
b = q;
c = beta;
th_c = theta_c;
fwdkin = [0 0 0 0 0 0];
fwdkin(1) =a;
fwdkin(2) =b;
fwdkin(3) =c;
fwdkin(4) =x_c;
fwdkin(5) =y_c;
fwdkin(6) =th_c;

== matlab function chris_3R_setpoint/Cluster_Controller1/Cluster Velocities to Cartesian Velocities ==
  data: fwdkin input; xc_err input; x1 output; zc_err input; thC_err input; a_err input; b_err input; C_err input; z1 output; th1 output; x2 output; z2 output; th2 output; x3 output; z3 output; th3 output
function [x1, z1,th1, x2,z2,th2, x3,z3, th3] = InverseJabobian(fwdkin, xc_err, zc_err, thC_err, a_err, b_err, C_err)
%% Unpacking the information from fwd_kin
p = fwdkin(1);
q = fwdkin(2);
beta = fwdkin(3);
xc = fwdkin(4);
yc = fwdkin(5);
theta_c = fwdkin(6);
yc_err = zc_err;
theta_c_err = thC_err;
p_err = a_err;
q_err = b_err;
beta_err = C_err;
%% Inverse Kinematics
  % Calculate x1, y1, and theta1 (Equations 12, 13, and 14)
r = sqrt((q + p*cos(beta))^2 + (p*sin(beta))^2);
  
x1 = xc + (1/3)*r*sin(theta_c);
y1 = yc + (1/3)*r*cos(theta_c);
%theta1 = phi1 - theta_c;
% Calculate x2, y2, and theta2 (Equations 15, 16, and 17)
x2 = xc + (1/3)*r*sin(theta_c) - p*sin(beta/2 + theta_c);
y2 = yc + (1/3)*r*cos(theta_c) - p*cos(beta/2 + theta_c);
%theta2 = phi2 - theta_c;
% Calculate x3, y3, and theta3 (Equations 18, 19, and 20)
x3 = xc + (1/3)*r*sin(theta_c) + q*sin(beta/2 - theta_c);
y3 = yc + (1/3)*r*cos(theta_c) - q*cos(beta/2 - theta_c);
%theta3 = phi3 - theta_c;
%% Now to take the partial derivates
% syms p q beta xc yc theta_c p_err q_err beta_err xc_err yc_err theta_c_err
% 
% % Define the equations
% eqs = [
%   xc + (1/3)*(sqrt((q + p*cos(beta))^2 + (p*sin(beta))^2))*sin(theta_c); % x1
%   yc + (1/3)*(sqrt((q + p*cos(beta))^2 + (p*sin(beta))^2))*cos(theta_c); % y1
%   xc + (1/3)*(sqrt((q + p*cos(beta))^2 + (p*sin(beta))^2))*sin(theta_c) - p*sin(beta/2 + theta_c); % x2
%   yc + (1/3)*(sqrt((q + p*cos(beta))^2 + (p*sin(beta))^2))*cos(theta_c) - p*cos(beta/2 + theta_c); % y2
%   xc + (1/3)*(sqrt((q + p*cos(beta))^2 + (p*sin(beta))^2))*sin(theta_c) + q*sin(beta/2 - theta_c); % x3
%   yc + (1/3)*(sqrt((q + p*cos(beta))^2 + (p*sin(beta))^2))*cos(theta_c) - q*cos(beta/2 - theta_c)  % y3
% ];
% 
% % Define the variables for differentiation
% vars = [p, q, beta, xc, yc, theta_c];
% 
% % Define the errors
% errs = [p_err, q_err, beta_err, xc_err, yc_err, theta_c_err];
% 
% % Initialize an array to store the sums (as symbolic)
% sums = sym(zeros(length(eqs), 1));
% 
% % Loop through equations and variables
% for i = 1:length(eqs)
%   for j = 1:length(vars)
%     derivative = diff(eqs(i), vars(j));
%     sums(i) = sums(i) + derivative * errs(j);
%   end
% end
% 
% % Display the results
% disp(simplify(sums(1)))
% disp(simplify(sums(2)))
% disp(simplify(sums(3)))
% disp(simplify(sums(4)))
% disp(simplify(sums(5)))
% disp(simplify(sums(6)))
%% Now to sum it all up
x1 =(3*xc_err*(p^2 + 2*cos(beta)*p*q + q^2)^(1/2) + p*p_err*sin(theta_c) + q*q_err*sin(theta_c) + p^2*theta_c_err*cos(theta_c) + q^2*theta_c_err*cos(theta_c) + p*q_err*cos(beta)*sin(theta_c) + p_err*q*cos(beta)*sin(theta_c) + 2*p*q*theta_c_err*cos(beta)*cos(theta_c) - beta_err*p*q*sin(beta)*sin(theta_c))/(3*(p^2 + 2*cos(beta)*p*q + q^2)^(1/2));
 
z1 = (3*yc_err*(p^2 + 2*cos(beta)*p*q + q^2)^(1/2) + p*p_err*cos(theta_c) + q*q_err*cos(theta_c) - p^2*theta_c_err*sin(theta_c) - q^2*theta_c_err*sin(theta_c) + p*q_err*cos(beta)*cos(theta_c) + p_err*q*cos(beta)*cos(theta_c) - beta_err*p*q*sin(beta)*cos(theta_c) - 2*p*q*theta_c_err*cos(beta)*sin(theta_c))/(3*(p^2 + 2*cos(beta)*p*q + q^2)^(1/2));
 
x2 = xc_err - p_err*(sin(beta/2 + theta_c) - (sin(theta_c)*(p + q*cos(beta)))/(3*(p^2 + 2*cos(beta)*p*q + q^2)^(1/2))) - beta_err*((p*cos(beta/2 + theta_c))/2 + (p*q*sin(beta)*sin(theta_c))/(3*(p^2 + 2*cos(beta)*p*q + q^2)^(1/2))) + theta_c_err*((cos(theta_c)*(p^2 + 2*cos(beta)*p*q + q^2)^(1/2))/3 - p*cos(beta/2 + theta_c)) + (q_err*sin(theta_c)*(q + p*cos(beta)))/(3*(p^2 + 2*cos(beta)*p*q + q^2)^(1/2));
 
z2 = yc_err - p_err*(cos(beta/2 + theta_c) - (cos(theta_c)*(p + q*cos(beta)))/(3*(p^2 + 2*cos(beta)*p*q + q^2)^(1/2))) + beta_err*((p*sin(beta/2 + theta_c))/2 - (p*q*sin(beta)*cos(theta_c))/(3*(p^2 + 2*cos(beta)*p*q + q^2)^(1/2))) - (theta_c_err*sin(theta_c)*(p^2 + 2*cos(beta)*p*q + q^2)^(1/2))/3 + p*theta_c_err*sin(beta/2 + theta_c) + (q_err*cos(theta_c)*(q + p*cos(beta)))/(3*(p^2 + 2*cos(beta)*p*q + q^2)^(1/2));
 
x3 = xc_err + q_err*(sin(beta/2 - theta_c) + (sin(theta_c)*(q + p*cos(beta)))/(3*(p^2 + 2*cos(beta)*p*q + q^2)^(1/2))) + beta_err*((q*cos(beta/2 - theta_c))/2 - (p*q*sin(beta)*sin(theta_c))/(3*(p^2 + 2*cos(beta)*p*q + q^2)^(1/2))) + (theta_c_err*cos(theta_c)*(p^2 + 2*cos(beta)*p*q + q^2)^(1/2))/3 - q*theta_c_err*cos(beta/2 - theta_c) + (p_err*sin(theta_c)*(p + q*cos(beta)))/(3*(p^2 + 2*cos(beta)*p*q + q^2)^(1/2));
 
z3 = yc_err - theta_c_err*(q*sin(beta/2 - theta_c) + (sin(theta_c)*(p^2 + 2*cos(beta)*p*q + q^2)^(1/2))/3) - q_err*(cos(beta/2 - theta_c) - (cos(theta_c)*(q + p*cos(beta)))/(3*(p^2 + 2*cos(beta)*p*q + q^2)^(1/2))) + beta_err*((q*sin(beta/2 - theta_c))/2 - (p*q*sin(beta)*cos(theta_c))/(3*(p^2 + 2*cos(beta)*p*q + q^2)^(1/2))) + (p_err*cos(theta_c)*(p + q*cos(beta)))/(3*(p^2 + 2*cos(beta)*p*q + q^2)^(1/2));
 
th1 = 0;
th2 = 0;
th3 = 0;

== matlab function chris_3R_setpoint/Robot_signal_processing_1/Global to Body Rotation Matrix ==
  data: u input; y output
function y = fcn(u)

y = [cos(u) -sin(u) 0; sin(u) cos(u) 0; 0 0 1];
